simulink model "hexa_tilted_FxTESO_ANSFT"  (R2023a)
settings: Solver=ode4  StartTime=0.0  StopTime=72  FixedStep=0.01  RelTol=1e-3
model workspace (MAT data in the model file):
  hover_2m = [0  0  0  0  0  0; 0  0  0  0  0  0; 2  2  2  2  2  2; 0  0  0  0  0  0; 0  0  0  0  0  0; 0  0  0  0  0  0]
  square = [0  0  0  0  0  0; 0  0  0  0  0  0; 2.5  2.5  2.5  2.5  2.5  0; 0  0  0  0  0  0; 0  0  0  0  0  0; 0  0  0  0  0  0]
  tf = Simulink.Parameter
  tf.Value = 60
  tf.DataType = 'auto'
  tf.Complexity = 'real'
  tf.Dimensions = [1 1]
  tray0 = [0  0  0  0  0  0; 0  0  0  0  0  0; 0  5  5  5  5  0; 0  0  0  0  0  0; 0  0  0  0  0  0; 0  0  0  0  0  0]
  tray1 = [0  0  0  0  0  0; 0  0  0  0  0  0; 0  5  2.5  5  2.5  0; 0  0  0  0  0  0; 0  0  0  0  0  0; 0  0  0  0  0  0]
  tray2 = [0  2  2  -2  -2  0; 0  0  -2  -2  2  0; 0  5  2.5  5  2.5  0; 0  0  0  0  0  0; 0  0  0  0  0  0; 0  0  0  0  0  0]
  tray3 = [0  2  2  -2  -2  0; 0  0  -2  -2  2  0; 0  2.5  2.5  2.5  2.5  0; 0  0  0  0  0  0; 0  0  0  0  0  0; 0  0  0.785  0.785  0.785  0]
  tray4 = [0  2  2  -2  -2  0; 0  0  -2  -2  2  0; 0  5  2.5  5  2.5  0; 0  0.15  0.15  0.15  0.15  0; 0  0  0  0  0  0; 0  0  0.785  1.57  0.785  0]
  tray5 = [0  0  0  0  0  0; 0  0  0  0  0  0; 0  5  2.5  5  2.5  0; 0  0.15  0.15  0  0  0; 0  0  0.15  0.15  0  0; 0  0  0  0  0  0]
  tray_xyaw = [0  0  2  2  2  2; 0  0  0  0  0  0; 0  2.5  2.5  2.5  2.5  2.5; 0  0  0  0  0  0; 0  0  0  0  0  0; 1.57079632679  1.57079632679  1.57079632679  1.57079632679  1.57079632679  1.57079632679]
  tray_yaw = [0  0  0  0  0  0; 0  0  0  0  0  0; 0  2.5  5  2.5  0  2.5; 0  0  0  0  0  0; 0  0  0  0  0  0; 0  0  0.785  1.57  0.785  0]
undefined symbols (not defined in the file or in its folder): F, Light, MIL
libraries: dspsrcs4 x6, simulink x5, sharedtransform x2, robotcorelib x1, aerolibwind2 x1, SignalEditorBlockLib x1, uavutilslib x1
settings Model: Creator=adan  LastModifiedBy=adan
settings OptimizationCC: DefaultParameterBehavior=Inlined  EnhancedBackFolding=on  PassReuseOutputArgsAs=Individual arguments  ZeroExternalMemoryAtStartup=off  ZeroInternalMemoryAtStartup=off  OptimizeBlockOrder=speed  DifferentSizesBufferReuse=on  OptimizationCustomize=off  EfficientTunableParamExpr=on
settings DebuggingCC: ParameterTunabilityLossMsg=error
settings SFSimCC: MATLABDynamicMemAlloc=off
settings RTWCC: Description=Embedded Coder  SystemTargetFile=ert.tlc  TemplateMakefile=ert_default_tmf
settings CodeAppCC: ForceParamTrailComments=on  IgnoreCustomStorageClasses=off  OperatorAnnotations=on  SimulinkDataObjDesc=on  SFDataObjDesc=on  InsertBlockDesc=on
settings ERTTargetCC: TargetLangStandard=C99 (ISO)  GenerateSampleERTMain=on  InlinedParameterPlacement=NonHierarchical  ERTCustomFileTemplate=example_file_process.tlc

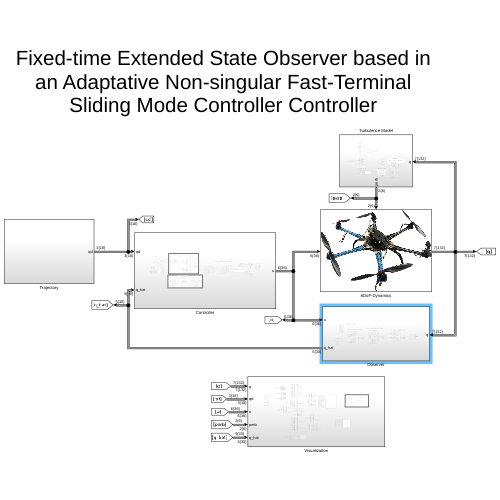
[thumbnail: Simulink's stored preview of the top-level diagram]
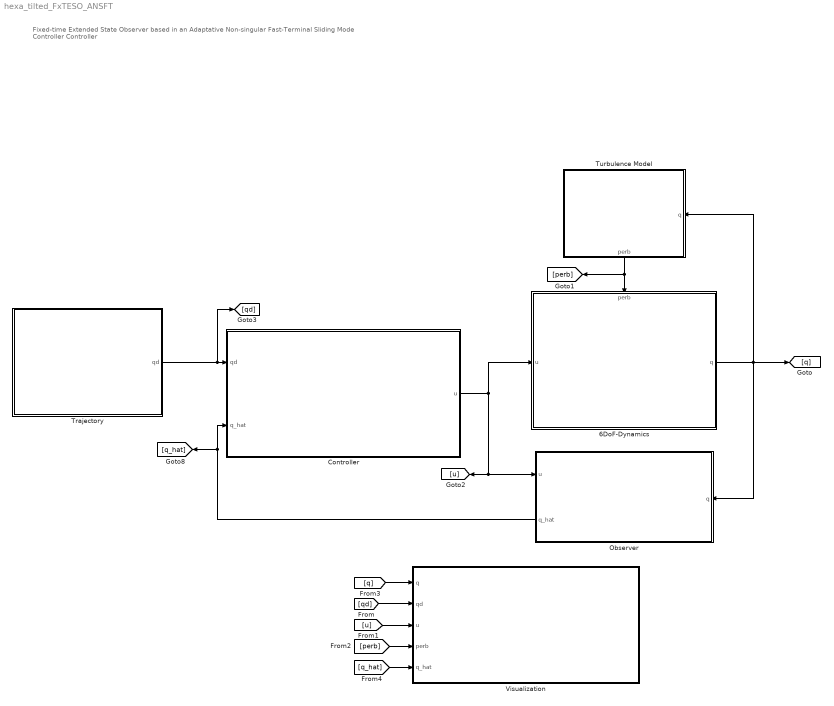
== system hexa_tilted_FxTESO_ANSFT ==
  note: Fixed-time Extended State Observer based in an Adaptative Non-singular Fast-Terminal Sliding Mode Controller Controller
  6DoF-Dynamics : Subsystem
      settings: PortSchema="{\"entries\":[{\"content\":{\"sides\":[{\"content\":{\"connectorIds\":[\"In1\"]},\"type\":\"ConnectorPlacement.EquallySpacedRectSide\",\"uuid\":\"d79ec49c-5563-41e0-ac59-6e897bc19fda\"},{\"content\":{\"connectorIds\":[\"Out1\"],\"side\":\"RIGHT\"},\"type\":\"ConnectorPlacement.EquallySpacedRectSide\",\"uuid\":\"1255043e-c90e-4bae-9fb4-4fa06f36f53e\"},{\"content\":{\"connectorIds\":[\"In2\"],\"side\":\"TOP\"},\"type\":\"ConnectorPlacement.EquallySpacedRectSide\",\"uuid\":\"823ada36-3f22-4ee3-87a1-180276f622bc\"}]},\"type\":\"ConnectorPlacement.EquallySpacedConnector\",\"uuid\":\"7403b609-b333-4977-a854-ed7a71f74338\"}],\"packageUris\":[\"http://schema.mathworks.com/mf0/Connector/R2020b\"],\"version\":\"1.0\"}"
      mask Display: image('$imagefile'); % Use "Edit Image" on toolstrip to change.
  Controller : Subsystem
  Observer : Subsystem
      settings: PortSchema="{\"entries\":[{\"content\":{\"sides\":[{\"content\":{\"connectorIds\":[\"In1\",\"Out1\"]},\"type\":\"ConnectorPlacement.EquallySpacedRectSide\",\"uuid\":\"d79ec49c-5563-41e0-ac59-6e897bc19fda\"},{\"content\":{\"connectorIds\":[\"In2\"],\"side\":\"RIGHT\"},\"type\":\"ConnectorPlacement.EquallySpacedRectSide\",\"uuid\":\"1255043e-c90e-4bae-9fb4-4fa06f36f53e\"},{\"content\":{\"side\":\"TOP\"},\"type\":\"ConnectorPlacement.EquallySpacedRectSide\",\"uuid\":\"823ada36-3f22-4ee3-87a1-180276f622bc\"}]},\"type\":\"ConnectorPlacement.EquallySpacedConnector\",\"uuid\":\"7403b609-b333-4977-a854-ed7a71f74338\"}],\"packageUris\":[\"http://schema.mathworks.com/mf0/Connector/R2020b\"],\"version\":\"1.0\"}"
  Trajectory : Subsystem
  Turbulence Model : Subsystem
      settings: PortSchema="{\"entries\":[{\"content\":{\"sides\":[{\"content\":{},\"type\":\"ConnectorPlacement.EquallySpacedRectSide\",\"uuid\":\"1a11629b-61d3-4a8e-8df8-8509e014e579\"},{\"content\":{\"connectorIds\":[\"In1\"],\"side\":\"RIGHT\"},\"type\":\"ConnectorPlacement.EquallySpacedRectSide\",\"uuid\":\"4b15c564-9714-4da5-9436-a08c0d95800f\"},{\"content\":{\"side\":\"TOP\"},\"type\":\"ConnectorPlacement.EquallySpacedRectSide\",\"uuid\":\"dd21b825-2def-4360-b27b-b8c6f475bfab\"},{\"content\":{\"connectorIds\":[\"Out1\"],\"side\":\"BOTTOM\"},\"type\":\"ConnectorPlacement.EquallySpacedRectSide\",\"uuid\":\"280c85e9-e29e-4357-9b86-73bf90833918\"}]},\"type\":\"ConnectorPlacement.EquallySpacedConnector\",\"uuid\":\"4c6e67eb-825c-4dd0-a48b-2afa68ae74f5\"}],\"packageUris\":[\"http://schema.mathworks.com/mf0/Connector/R2020b\"],\"version\":\"1.0\"}"
  Visualization : Subsystem
  wires:
  Trajectory/1(qd) -> [qd], Controller/1(qd)
  Controller/1(u) -> 6DoF-Dynamics/1(u), [u], Observer/1(u)
  6DoF-Dynamics/1(q) -> Turbulence Model/1(q), [q], Observer/2(q)
  Turbulence Model/1(perb) -> 6DoF-Dynamics/2(perb), [perb]
  Observer/1(q_hat) -> [q_hat], Controller/2(q_hat)
  [qd] -> Visualization/2(qd)
  [u] -> Visualization/3(u)
  [perb] -> Visualization/4(perb)
  [q_hat] -> Visualization/5(q_hat)
  [q] -> Visualization/1(q)

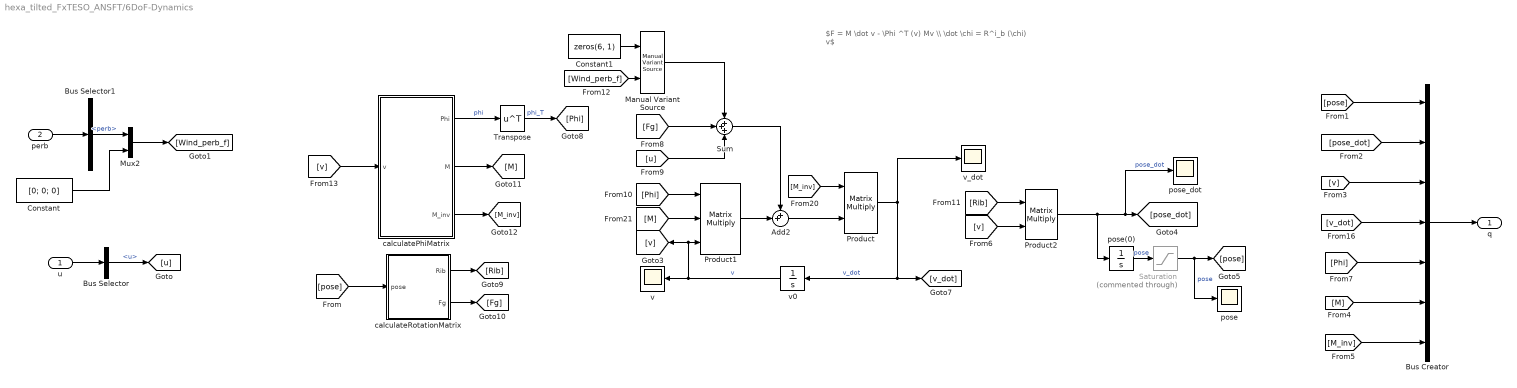
== system hexa_tilted_FxTESO_ANSFT/6DoF-Dynamics ==
  note: $F = M \dot v - \Phi ^T (v) Mv \\ \dot \chi = R^i_b (\chi) v$
  u : Inport
  perb : Inport  Port=2
  Add2 : Sum  Inputs=++|
  Bus Creator : BusCreator  Inputs=7
  Bus Selector : BusSelector  OutputSignals=u
  Bus Selector1 : BusSelector  OutputSignals=perb
  Constant : Constant  Value=[0; 0; 0]
  Constant1 : Constant  Value=zeros(6, 1)
  Manual Variant Source : simulink/Signal Routing/Manual Variant Source  NumChoices=2  LabelModeActiveChoice=V_2
  Mux2 : Mux  Inputs=2
  Product : Product  Multiplication=Matrix(*)
  Product1 : Product  Inputs=3  Multiplication=Matrix(*)
  Product2 : Product  Multiplication=Matrix(*)
  Saturation : Saturate  Commented=through  UpperLimit=[10, 10, 10, 10, 10, 10]'  LowerLimit=[-10, -10, 0, -10, -10, -10]'
  Sum : Sum  Inputs=+++
  Transpose : Math  Operator=transpose
  calculatePhiMatrix : MATLAB Function  TreatAsAtomicUnit=on
  calculateRotationMatrix : MATLAB Function  TreatAsAtomicUnit=on
  pose : Scope
  pose(0) : Integrator  InitialCondition=[0; 0; 0; 0; 0; 0]
  pose_dot : Scope
  v : Scope
  v0 : Integrator  InitialCondition=[0; 0; 0; 0; 0; 0]
  v_dot : Scope
  q : Outport
  wires:
  [M_inv] -> Product/1
  Product1/1 -> Add2/2
  [v] -> Product2/2
  Add2/1 -> Product/2
  Product/1 -> v_dot/1, [v_dot], v0/1  "v_dot"
  Product2/1 -> pose(0)/1, pose_dot/1, [pose_dot]  "pose_dot"
  [M] -> Product1/2
  [Rib] -> Product2/1
  [Phi] -> Product1/1
  [v] -> calculatePhiMatrix/1(v)
  calculatePhiMatrix/2(M) -> [M]
  calculatePhiMatrix/1(Phi) -> Transpose/1  "phi"
  calculatePhiMatrix/3(M_inv) -> [M_inv]
  Transpose/1 -> [Phi]  "phi_T"
  calculateRotationMatrix/1(Rib) -> [Rib]
  calculateRotationMatrix/2(Fg) -> [Fg]
  [pose] -> calculateRotationMatrix/1(pose)
  u/1 -> Bus Selector/1
  [pose] -> Bus Creator/1
  [pose_dot] -> Bus Creator/2
  [v] -> Bus Creator/3
  Bus Creator/1 -> q/1
  [Phi] -> Bus Creator/5
  [M] -> Bus Creator/6
  [M_inv] -> Bus Creator/7
  [Fg] -> Sum/2
  perb/1 -> Bus Selector1/1
  Bus Selector/1 -> [u]  "<u>"
  [u] -> Sum/3
  Bus Selector1/1 -> Mux2/1  "<perb>"
  Constant/1 -> Mux2/2
  Mux2/1 -> [Wind_perb_f]
  [Wind_perb_f] -> Manual Variant Source/2
  Sum/1 -> Add2/1
  v0/1 -> [v], Product1/3, v/1  "v"
  pose(0)/1 -> Saturation/1  "pose"
  [v_dot] -> Bus Creator/4
  Saturation/1 -> [pose], pose/1  "pose"
  Constant1/1 -> Manual Variant Source/1
  Manual Variant Source/1 -> Sum/1

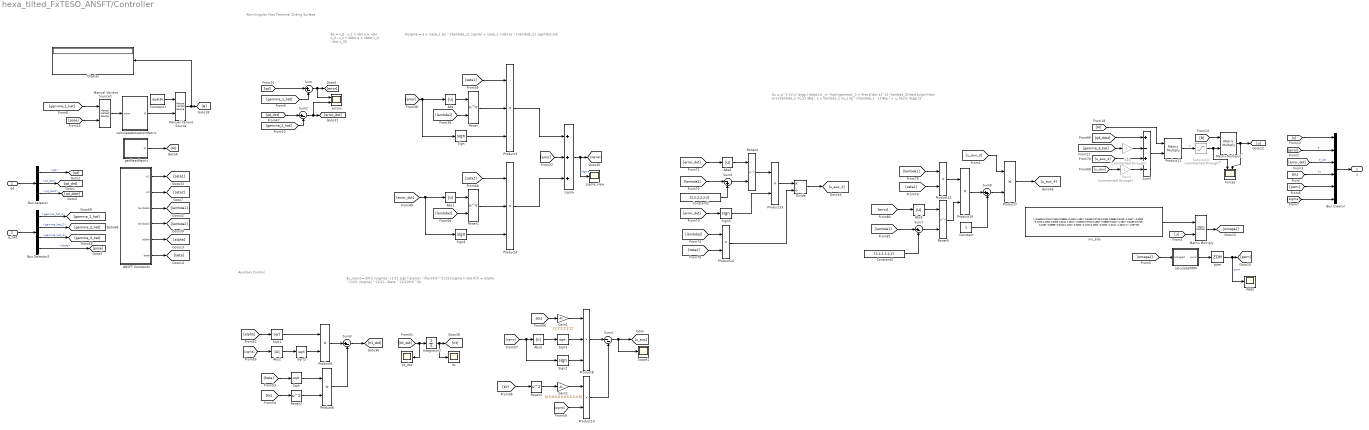
== system hexa_tilted_FxTESO_ANSFT/Controller ==
  note: $u = g^{-1}(x) \bigg [ \ddot{x}_d - \hat{\gamma}_3 + \frac{|\dot e|^{2- \lambda_2}\text{sign}(\dot e)}{\lambda_2 \xi_2} \Big ( 1 + \lambda_1 \xi_1 |e|^{\lambda_1 - 1}\Big ) + u_{aux} \bigg ]$
  note: Auxiliary Control
  note: Non-Singular Fast Terminal Sliding Surface
  note: $e = x_d - x_1 \\ \dot e = \dot x_d - x_2 \\ \ddot e = \ddot x_d - \dot x_2$
  note: $\sigma = e + \zeta_1 |e| ^{\lambda_1} sign(e) + \zeta_2 | \dot e| ^{\lambda_2} sign(\dot e)$
  note: $u_{aux}=-2K(t) |\sigma|^{1/2} sign (\sigma) - \frac{K(t)^2}{2}\sigma \\ \dot K(t) = \alpha ^{1/2} |\sigma| ^{1/2} - \beta ^{1/2}K(t)^2$
  qd : Inport
  q_hat : Inport  Port=2
  ANSFT Constants : MATLAB Function  TreatAsAtomicUnit=on
  Abs{,1..5} (6 alike) : Abs  SaturateOnIntegerOverflow=off
  Bus Creator : BusCreator  Inputs=6
  Bus Selector : BusSelector  OutputSignals=qd,qd_dot,qd_ddot
  Bus Selector2 : BusSelector  OutputSignals=gamma_hat_1,gamma_hat_2,gamma_hat_3,pose
  Constant : Constant
  Constant1 : Constant  Value=eye(6)
  Constant2 : Constant  Value=[2;2;2;2;2;2]
  Constant3 : Constant  Value=[1;1;1;1;1;1]
  Display : Display
  Divide : Product  Inputs=*/
  Forces : Scope  NumInputPorts=2
  Gain : Gain  Commented=through  Gain=-1
  Gain1 : Gain  Gain=[2;2;2;2;2;2]
  Gain2 : Gain  Gain=[0.5;0.5;0.5;0.5;0.5;0.5]
  Gain3 : Gain  Commented=through  Gain=-1
  Integrator2 : Integrator  InitialCondition=[0;0;0;0;0;0]
  Kt : Scope
  Kt_dot : Scope
  Manual Variant Source : simulink/Signal Routing/Manual Variant Source  NumChoices=2  LabelModeActiveChoice=V_2
  Manual Variant Source1 : simulink/Signal Routing/Manual Variant Source  NumChoices=2  LabelModeActiveChoice=V_2
  Matrix Multiply : Product  Multiplication=Matrix(*)
  Matrix Multiply1 : Product  Multiplication=Matrix(*)
  PWM : Scope
  Power{,1,4..5} (4 alike) : Math  Operator=pow
  Power2 : Math  Operator=square
  Power3 : Math  Operator=square
  Product{5..7,10,13..16} (8 alike) : Product
  Product11 : Product  Multiplication=Matrix(*)
  Product3 : Product  Inputs=3
  Product4 : Product  Inputs=3
  Product8 : Product  Inputs=3
  Saturation : Saturate  Commented=through  UpperLimit=[5, 5, 42, 0.5, 0.5, 0.5]'  LowerLimit=[-5, -5, 0, -0.5, -0.5, -0.5]'
  Scope1 : Scope
  Sign{,1..3} (4 alike) : Signum
  Sqrt{,1..3} (4 alike) : Sqrt
  Sum{,2..3,7} (4 alike) : Sum  Inputs=|+-
  Sum4 : Sum  Inputs=|--
  Sum5 : Sum  Inputs=+-+-
  Sum6 : Sum  Inputs=|-+
  Sum8 : Sum  Inputs=|++
  calculateActuationMatrix : MATLAB Function  TreatAsAtomicUnit=on
  calculatePWM : MATLAB Function  TreatAsAtomicUnit=on
  errors : Scope  NumInputPorts=2
  getMassMatrix : MATLAB Function  TreatAsAtomicUnit=on
  inv_allo : Constant  Value=|
      | [-0.6436    0.3716    0.1352    0.8869   -0.5120    1.1817;
      |             0.6436    0.3716    0.1352    0.8869    0.5120   -1.1817;
      |             -0.0000   -0.7431    0.1352    0.0000    1.0241    1.1817;
      |             -0.6436    0.3716    0.1352   -0.8869    0.5120   -1.1817;
      |             0.6436    0.3716    0.1352   -0.8869   -0.5120    1.1817;
      |             0.0000   -0.7431    0.1352   -0.0000   -1.0241   -1.1817;] * 1.0e+05;
  pwm : ZeroOrderHold  SampleTime=-1
  sigma : Sum  Inputs=+++
  sigma_view : Scope
  u : Outport
  wires:
  Product6/1 -> Sum3/2
  Sign1/1 -> Product4/3
  Sum8/1 -> Product7/2
  Product5/1 -> Sum3/1
  [error_dot] -> Abs4/1
  [u_aux_3] -> Product7/1
  Power5/1 -> Product16/2
  [zeta1] -> Product3/1
  Constant/1 -> Sum8/2
  Product16/1 -> Sum8/1
  Sqrt/1 -> Product6/1
  Product10/1 -> Sum4/2
  Sum6/1 -> Power4/2
  Product15/1 -> Product16/1
  [qd_ddot] -> Sum5/1
  [lambda2] -> Sum6/1
  Sum4/1 -> Scope1/1, [u_aux]
  [Kt] -> Power2/1
  Gain1/1 -> Product8/1
  Sum5/1 -> Product11/2
  Sqrt1/1 -> Product5/1
  Constant2/1 -> Sum6/2
  Sign3/1 -> Product13/2
  [lambda1] -> Sum7/1
  [gamma_2_hat] -> Sum2/2
  Power3/1 -> Gain2/1
  Product3/1 -> sigma/1
  [beta] -> Sqrt/1
  Abs4/1 -> Power4/1
  [Kt] -> Gain1/1
  [error_dot] -> Sign1/1, Abs1/1
  Divide/1 -> [u_aux_3]
  [sigma] -> Sign2/1, Abs3/1
  [zeta2] -> Product14/2
  Sum3/1 -> [Kt_dot]
  Product8/1 -> Sum4/1
  [sigma] -> Abs2/1
  Power/1 -> Product3/2
  Product4/1 -> sigma/3
  Constant3/1 -> Sum7/2
  [error] -> sigma/2
  Abs3/1 -> Sqrt3/1
  [alpha] -> Sqrt1/1
  Sum7/1 -> Power5/2
  Sqrt2/1 -> Product5/2
  Power4/1 -> Product13/1
  [M] -> Product11/1
  sigma/1 -> sigma_view/1, [sigma]  "sigma"
  Sign/1 -> Product3/3
  Abs2/1 -> Sqrt2/1
  [Kt_dot] -> Kt_dot/1, Integrator2/1
  Power1/1 -> Product4/2
  [lambda2] -> Product14/1
  Power2/1 -> Product6/2
  [zeta1] -> Product15/2
  [Kt] -> Power3/1
  [lambda1] -> Product15/1
  [error_dot] -> Sign3/1
  Sqrt3/1 -> Product8/2
  Product13/1 -> Divide/1
  [zeta2] -> Product4/1
  Integrator2/1 -> Kt/1, [Kt]
  [gamma_1_hat] -> Sum/2
  Abs/1 -> Power/1
  [qd] -> Sum/1
  Abs1/1 -> Power1/1
  Sum2/1 -> errors/2, [error_dot]
  Sum/1 -> errors/1, [error]
  Gain2/1 -> Product10/1
  Product14/1 -> Divide/2
  [lambda2] -> Power1/2
  [error] -> Abs5/1
  Abs5/1 -> Power5/1
  Product7/1 -> [u_aux_4]
  [sigma] -> Product10/2
  [lambda1] -> Power/2
  Sign2/1 -> Product8/3
  [error] -> Sign/1, Abs/1
  [qd_dot] -> Sum2/1
  Bus Creator/1 -> u/1
  ANSFT Constants/3(lambda1) -> [lambda1]
  ANSFT Constants/1(xi1) -> [zeta1]
  ANSFT Constants/2(xi2) -> [zeta2]
  ANSFT Constants/5(alpha) -> [alpha]
  ANSFT Constants/6(beta) -> [beta]
  ANSFT Constants/4(lambda2) -> [lambda2]
  qd/1 -> Bus Selector/1
  Bus Selector/2 -> [qd_dot]  "<qd_dot>"
  Bus Selector/1 -> [qd]  "<qd>"
  Bus Selector/3 -> [qd_ddot]  "<qd_ddot>"
  Product11/1 -> Saturation/1  "u"
  [error] -> Bus Creator/2  "e"
  [error_dot] -> Bus Creator/3  "e_dot"
  [Kt] -> Bus Creator/4  "kt"
  inv_allo/1 -> Matrix Multiply/1
  [u] -> Matrix Multiply/2
  Matrix Multiply/1 -> [omega2]
  [omega2] -> calculatePWM/1(omega2)
  calculatePWM/1(pwm) -> pwm/1
  pwm/1 -> PWM/1, [pwm]  "pwm"
  [pwm] -> Bus Creator/5
  [sigma] -> Bus Creator/6
  q_hat/1 -> Bus Selector2/1
  Bus Selector2/2 -> [gamma_2_hat]  "<gamma_hat_2>"
  Bus Selector2/3 -> [gamma_3_hat]  "<gamma_hat_3>"
  Bus Selector2/1 -> [gamma_1_hat]  "<gamma_hat_1>"
  [gamma_3_hat] -> Gain/1
  [u] -> Bus Creator/1
  Saturation/1 -> Matrix Multiply1/2, Forces/1  "u"
  getMassMatrix/1(M) -> [M]
  [u_aux_4] -> Sum5/3
  [u_aux] -> Gain3/1
  Gain/1 -> Sum5/2
  Gain3/1 -> Sum5/4
  calculateActuationMatrix/1(B) -> Manual Variant Source/2
  [gamma_1_hat] -> Manual Variant Source1/1
  Matrix Multiply1/1 -> Forces/2, [u]  "u"
  [B] -> Matrix Multiply1/1
  Manual Variant Source/1 -> Display/1, [B]
  Constant1/1 -> Manual Variant Source/1
  Bus Selector2/4 -> [pose]  "<pose>"
  Manual Variant Source1/1 -> calculateActuationMatrix/1(pose)
  [pose] -> Manual Variant Source1/2

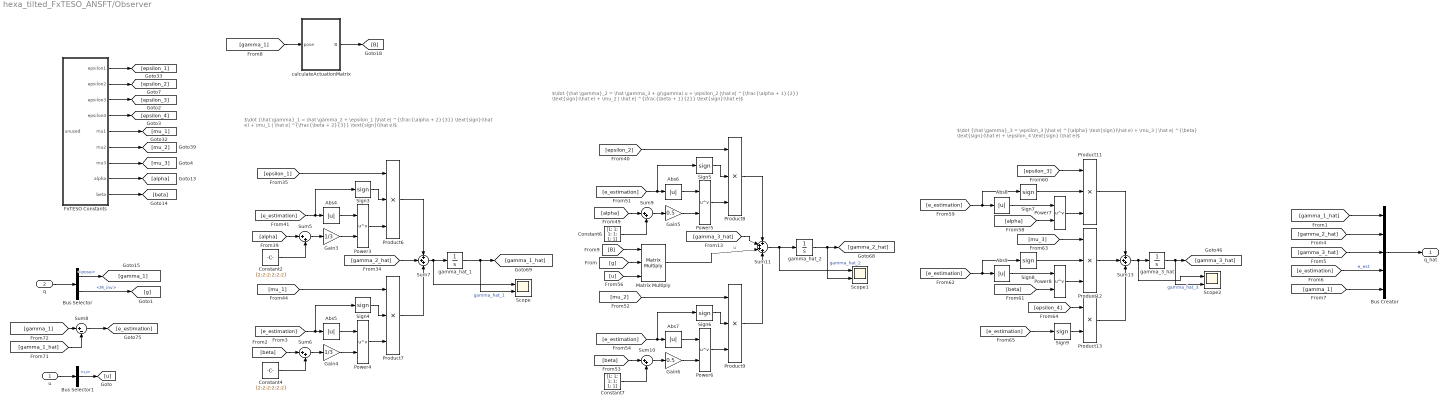
== system hexa_tilted_FxTESO_ANSFT/Observer ==
  note: $\dot {\hat \gamma}_3 = \epsilon_3 |\hat e| ^{\alpha} \text{sign}(\hat e) + \mu_3 | \hat e| ^{\beta} \text{sign}(\hat e) + \epsilon_4 \text{sign} (\hat e)$
  note: $\dot {\hat \gamma}_1 = \hat \gamma_2 + \epsilon_1 |\hat e| ^{\frac{\alpha + 2}{3}} \text{sign}(\hat e) + \mu_1 | \hat e| ^{\frac{\beta + 2}{3}} \text{sign}(\hat e)$
  note: $\dot {\hat \gamma}_2 = \hat \gamma_3 + g(\gamma) u + \epsilon_2 |\hat e| ^{\frac{\alpha + 1}{2}} \text{sign}(\hat e) + \mu_2 | \hat e| ^{\frac{\beta + 1}{2}} \text{sign}(\hat e)$
  u : Inport
  q : Inport  Port=2
  Abs{4..9} (6 alike) : Abs  SaturateOnIntegerOverflow=off
  Bus Creator : BusCreator  Inputs=5
  Bus Selector : BusSelector  OutputSignals=pose,M_inv
  Bus Selector1 : BusSelector  OutputSignals=u
  Constant2 : Constant  Value=[2;2;2;2;2;2]
  Constant4 : Constant  Value=[2;2;2;2;2;2]
  Constant6 : Constant  Value=[1; 1; 1; 1; 1; 1]
  Constant7 : Constant  Value=[1; 1; 1; 1; 1; 1]
  FxTESO Constants : MATLAB Function  TreatAsAtomicUnit=on
  Gain3 : Gain  Gain=1/3
  Gain4 : Gain  Gain=1/3
  Gain5 : Gain  Gain=0.5
  Gain6 : Gain  Gain=0.5
  Matrix Multiply : Product  Inputs=3  Multiplication=Matrix(*)
  Power{3..8} (6 alike) : Math  Operator=pow
  Product{6..9,11..12} (6 alike) : Product  Inputs=3
  Product13 : Product
  Scope : Scope  NumInputPorts=2
  Scope1 : Scope  NumInputPorts=2
  Scope2 : Scope  NumInputPorts=2
  Sign{3..9} (7 alike) : Signum
  Sum{5..6,9..10} (4 alike) : Sum  Inputs=|++
  Sum11 : Sum  Inputs=++++
  Sum13 : Sum  Inputs=+++
  Sum7 : Sum  Inputs=+++
  Sum8 : Sum  Inputs=|+-
  calculateActuationMatrix : MATLAB Function  TreatAsAtomicUnit=on
  gamma_3_hat : Integrator  InitialCondition=[0; 0; -9.81; 0; 0; 0]
  gamma_hat_1 : Integrator  InitialCondition=[0; 0; 0; 0; 0; 0]
  gamma_hat_2 : Integrator  InitialCondition=zeros(6,1)
  q_hat : Outport
  wires:
  [gamma_1] -> Sum8/1
  Gain6/1 -> Power6/2
  [alpha] -> Power7/2
  [gamma_3_hat] -> Sum11/2
  Sign7/1 -> Product11/2
  Sum7/1 -> Scope/1, gamma_hat_1/1
  Abs7/1 -> Power6/1
  [gamma_1_hat] -> Sum8/2
  [alpha] -> Sum5/1
  Sum8/1 -> [e_estimation]
  Power4/1 -> Product7/3
  [epsilon_3] -> Product11/1
  Power3/1 -> Product6/3
  Constant2/1 -> Sum5/2
  Abs9/1 -> Power8/1
  Sign5/1 -> Product8/2
  [e_estimation] -> Abs9/1, Sign8/1
  Gain4/1 -> Power4/2
  [e_estimation] -> Sign5/1, Abs6/1
  [mu_3] -> Product12/1
  Power7/1 -> Product11/3
  [beta] -> Power8/2
  Sign8/1 -> Product12/2
  [epsilon_1] -> Product6/1
  Bus Selector/1 -> [gamma_1]  "<pose>"
  Product13/1 -> Sum13/3
  Sign9/1 -> Product13/2
  Sum11/1 -> Scope1/1, gamma_hat_2/1
  Sum5/1 -> Gain3/1
  Product7/1 -> Sum7/3
  [e_estimation] -> Sign6/1, Abs7/1
  Abs4/1 -> Power3/1
  Abs8/1 -> Power7/1
  [e_estimation] -> Sign4/1, Abs5/1
  Sum9/1 -> Gain5/1
  [e_estimation] -> Abs8/1, Sign7/1
  Sum13/1 -> Scope2/1, gamma_3_hat/1
  [e_estimation] -> Sign3/1, Abs4/1
  Sign6/1 -> Product9/2
  [beta] -> Sum10/1
  Power8/1 -> Product12/3
  Sign3/1 -> Product6/2
  [mu_1] -> Product7/1
  [mu_2] -> Product9/1
  [gamma_2_hat] -> Sum7/2
  [epsilon_4] -> Product13/1
  [beta] -> Sum6/1
  Sum10/1 -> Gain6/1
  Gain3/1 -> Power3/2
  Constant4/1 -> Sum6/2
  gamma_hat_1/1 -> Scope/2, [gamma_1_hat]  "gamma_hat_1"
  [epsilon_2] -> Product8/1
  Abs5/1 -> Power4/1
  Sign4/1 -> Product7/2
  Gain5/1 -> Power5/2
  Product12/1 -> Sum13/2
  gamma_hat_2/1 -> Scope1/2, [gamma_2_hat]  "gamma_hat_2"
  Product6/1 -> Sum7/1
  [e_estimation] -> Sign9/1
  Product8/1 -> Sum11/1
  Constant6/1 -> Sum9/2
  [alpha] -> Sum9/1
  Abs6/1 -> Power5/1
  Power6/1 -> Product9/3
  Product11/1 -> Sum13/1
  Constant7/1 -> Sum10/2
  gamma_3_hat/1 -> Scope2/2, [gamma_3_hat]  "gamma_hat_3"
  Sum6/1 -> Gain4/1
  Power5/1 -> Product8/3
  Matrix Multiply/1 -> Sum11/3  "u"
  Product9/1 -> Sum11/4
  FxTESO Constants/5(mu1) -> [mu_1]
  FxTESO Constants/1(epsilon1) -> [epsilon_1]
  FxTESO Constants/2(epsilon2) -> [epsilon_2]
  FxTESO Constants/8(alpha) -> [alpha]
  FxTESO Constants/9(beta) -> [beta]
  FxTESO Constants/6(mu2) -> [mu_2]
  q/1 -> Bus Selector/1
  Bus Selector/2 -> [g]  "<M_inv>"
  FxTESO Constants/4(epsilon4) -> [epsilon_4]
  FxTESO Constants/3(epsilon3) -> [epsilon_3]
  FxTESO Constants/7(mu3) -> [mu_3]
  u/1 -> Bus Selector1/1
  Bus Selector1/1 -> [u]  "<u>"
  [gamma_1_hat] -> Bus Creator/1
  [gamma_3_hat] -> Bus Creator/3
  [gamma_2_hat] -> Bus Creator/2
  Bus Creator/1 -> q_hat/1
  [e_estimation] -> Bus Creator/4  "e_est"
  [gamma_1] -> Bus Creator/5
  [gamma_1] -> calculateActuationMatrix/1(pose)
  calculateActuationMatrix/1(B) -> [B]
  [B] -> Matrix Multiply/1
  [g] -> Matrix Multiply/2
  [u] -> Matrix Multiply/3

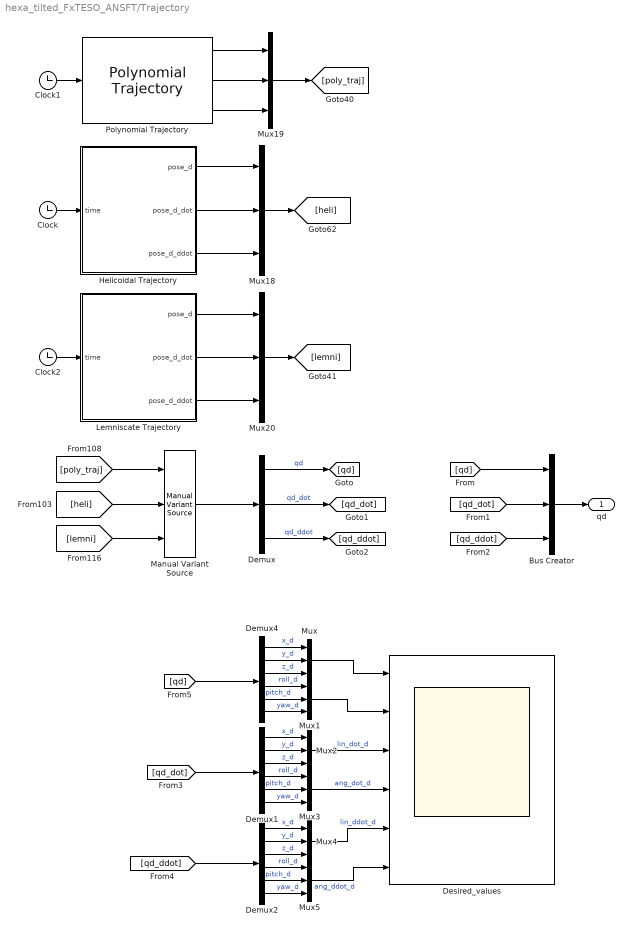
== system hexa_tilted_FxTESO_ANSFT/Trajectory ==
  Bus Creator : BusCreator  Inputs=3
  Clock : Clock
  Clock1 : Clock
  Clock2 : Clock
  Demux : Demux  Outputs=3
  Demux1 : Demux  Outputs=6
  Demux2 : Demux  Outputs=6
  Demux4 : Demux  Outputs=6
  Desired_values : Scope  NumInputPorts=6
  Helicoidal Trajectory : MATLAB Function  TreatAsAtomicUnit=on
  Lemniscate Trajectory : MATLAB Function  TreatAsAtomicUnit=on
  Manual Variant Source : simulink/Signal Routing/Manual Variant Source  NumChoices=3  LabelModeActiveChoice=V_2
  Mux{,1..5,18..20} (9 alike) : Mux  Inputs=3
  Polynomial Trajectory : robotcorelib/Polynomial Trajectory  WaypointSource=Internal  Waypoints=tray_xyaw  TimePoints=[ 0, 12, 24, 36, 48, tf ]  TimeInterval=[ 1, 4 ]  Method=Cubic Polynomial  ParameterSource=Internal  VelocityBoundaryCondition=zeros( 6, 6 )  AccelerationBoundaryCondition=zeros( 2, 5 )  SimulateUsing=Interpreted execution
  qd : Outport
  wires:
  Manual Variant Source/1 -> Demux/1
  Lemniscate Trajectory/2(pose_d_dot) -> Mux20/2
  [poly_traj] -> Manual Variant Source/1
  Polynomial Trajectory/3 -> Mux19/3
  Helicoidal Trajectory/1(pose_d) -> Mux18/1
  Clock1/1 -> Polynomial Trajectory/1
  Mux18/1 -> [heli]
  Lemniscate Trajectory/3(pose_d_ddot) -> Mux20/3
  Polynomial Trajectory/2 -> Mux19/2
  Demux/2 -> [qd_dot]  "qd_dot"
  Clock2/1 -> Lemniscate Trajectory/1(time)
  Helicoidal Trajectory/3(pose_d_ddot) -> Mux18/3
  Demux/1 -> [qd]  "qd"
  Mux19/1 -> [poly_traj]
  Mux20/1 -> [lemni]
  Lemniscate Trajectory/1(pose_d) -> Mux20/1
  Helicoidal Trajectory/2(pose_d_dot) -> Mux18/2
  Clock/1 -> Helicoidal Trajectory/1(time)
  Demux/3 -> [qd_ddot]  "qd_ddot"
  [heli] -> Manual Variant Source/2
  [lemni] -> Manual Variant Source/3
  Bus Creator/1 -> qd/1
  Polynomial Trajectory/1 -> Mux19/1
  Demux4/4 -> Mux1/1  "roll_d"
  Demux4/6 -> Mux1/3  "yaw_d"
  Demux4/3 -> Mux/3  "z_d"
  Demux4/2 -> Mux/2  "y_d"
  Demux4/1 -> Mux/1  "x_d"
  Demux4/5 -> Mux1/2  "pitch_d"
  [qd] -> Bus Creator/1
  [qd_dot] -> Bus Creator/2
  [qd_ddot] -> Bus Creator/3
  Demux1/6 -> Mux3/3  "yaw_d"
  Demux1/3 -> Mux2/3  "z_d"
  Demux1/5 -> Mux3/2  "pitch_d"
  [qd_dot] -> Demux1/1
  Demux1/1 -> Mux2/1  "x_d"
  Demux1/4 -> Mux3/1  "roll_d"
  Demux1/2 -> Mux2/2  "y_d"
  Demux2/6 -> Mux5/3  "yaw_d"
  Demux2/3 -> Mux4/3  "z_d"
  Demux2/5 -> Mux5/2  "pitch_d"
  [qd_ddot] -> Demux2/1
  Demux2/1 -> Mux4/1  "x_d"
  Demux2/4 -> Mux5/1  "roll_d"
  Demux2/2 -> Mux4/2  "y_d"
  Mux/1 -> Desired_values/1
  Mux1/1 -> Desired_values/2
  Mux2/1 -> Desired_values/3  "lin_dot_d"
  Mux3/1 -> Desired_values/4  "ang_dot_d"
  Mux4/1 -> Desired_values/5  "lin_ddot_d"
  Mux5/1 -> Desired_values/6  "ang_ddot_d"
  [qd] -> Demux4/1

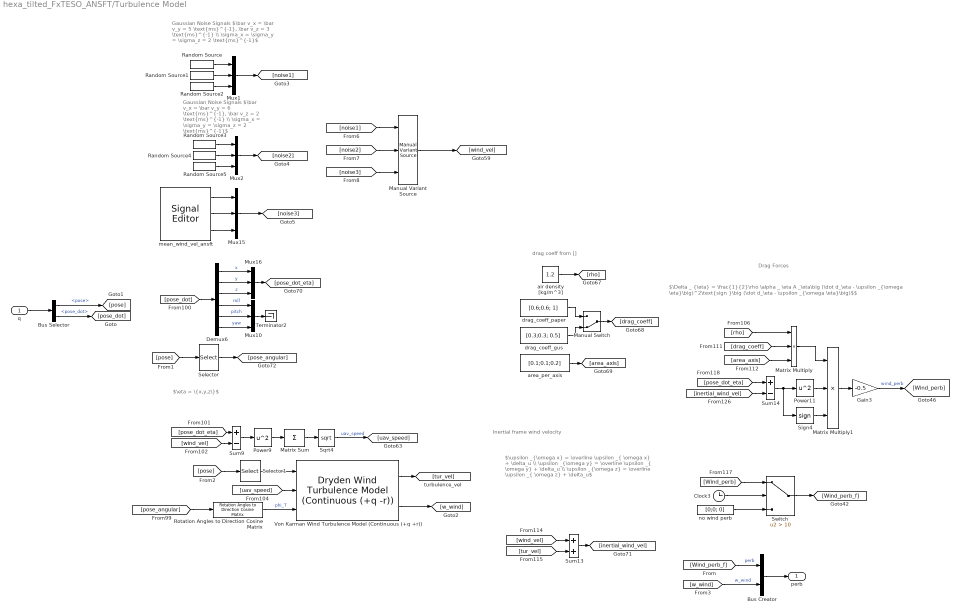
== system hexa_tilted_FxTESO_ANSFT/Turbulence Model ==
  note: $\Delta _ {\eta} = \frac{1}{2}\rho \alpha _ \eta A _\eta\big (\dot d_\eta - \upsilon _{\omega \eta}\big)^2\text{sign }\big (\dot d_\eta - \upsilon _{\omega \eta}\big)$$
  note: drag coeff from []
  note: $\upsilon _{\omega x} = \overline \upsilon _{ \omega x} + \delta_u \\ \upsilon _{\omega y} = \overline \upsilon _{ \omega y} + \delta_u \\ \upsilon _{\omega z} = \overline \upsilon _{ \omega z} + \delta_u$
  note: $\eta = \{x,y,z\}$
  note: Drag Forces
  note: Inertial frame wind velocity
  note: Gaussian Noise Signals
      | $\bar v_x = \bar v_y = 5 \text{ms}^{-1}, \bar v_z = 3 \text{ms}^{-1} \\ \sigma_x = \sigma_y = \sigma_z = 2 \text{ms}^{-1}$
  note: Gaussian Noise Signals
      | $\bar v_x = \bar v_y = 6 \text{ms}^{-1}, \bar v_z = 2 \text{ms}^{-1} \\ \sigma_x = \sigma_y = \sigma_z = 2 \text{ms}^{-1}$
  q : Inport
  Bus Creator : BusCreator  Inputs=2
  Bus Selector : BusSelector  OutputSignals=pose,pose_dot
  Clock3 : Clock
  Demux6 : Demux  Outputs=6
  Gain3 : Gain  Gain=-0.5
  Manual Variant Source : simulink/Signal Routing/Manual Variant Source  NumChoices=3  LabelModeActiveChoice=V_1
  Manual Switch : ManualSwitch  CurrentSetting=0
  Matrix Sum : Sum  Inputs=+
  Matrix Multiply : Product  Inputs=3
  Matrix Multiply1 : Product  Inputs=3
  Mux{1..2,10,15..16} (5 alike) : Mux  Inputs=3
  Power11 : Math  Operator=square
  Power9 : Math  Operator=square
  Random Source : dspsrcs4/Random Source  SrcType=Gaussian  NormMethod=Ziggurat  CltLength=12  MinVal=0  MaxVal=1  MeanVal=5  VarVal=2  RepMode=Not repeatable  rawSeed=1  IsInherit=off  SampMode=Discrete  SampTime=1  SampFrame=1  DataType=Double  OutComplex=Real  OutputFrames=off
  Random Source1 : dspsrcs4/Random Source  SrcType=Gaussian  NormMethod=Ziggurat  CltLength=12  MinVal=0  MaxVal=1  MeanVal=5  VarVal=2  RepMode=Not repeatable  rawSeed=1  IsInherit=off  SampMode=Discrete  SampTime=1  SampFrame=1  DataType=Double  OutComplex=Real  OutputFrames=off
  Random Source2 : dspsrcs4/Random Source  SrcType=Gaussian  NormMethod=Ziggurat  CltLength=12  MinVal=0  MaxVal=1  MeanVal=3  VarVal=2  RepMode=Not repeatable  rawSeed=1  IsInherit=off  SampMode=Discrete  SampTime=1  SampFrame=1  DataType=Double  OutComplex=Real  OutputFrames=off
  Random Source3 : dspsrcs4/Random Source  SrcType=Gaussian  NormMethod=Ziggurat  CltLength=12  MinVal=0  MaxVal=1  MeanVal=6  VarVal=2  RepMode=Not repeatable  rawSeed=1  IsInherit=off  SampMode=Discrete  SampTime=1  SampFrame=1  DataType=Double  OutComplex=Real  OutputFrames=off
  Random Source4 : dspsrcs4/Random Source  SrcType=Gaussian  NormMethod=Ziggurat  CltLength=12  MinVal=0  MaxVal=1  MeanVal=6  VarVal=2  RepMode=Not repeatable  rawSeed=1  IsInherit=off  SampMode=Discrete  SampTime=1  SampFrame=1  DataType=Double  OutComplex=Real  OutputFrames=off
  Random Source5 : dspsrcs4/Random Source  SrcType=Gaussian  NormMethod=Ziggurat  CltLength=12  MinVal=0  MaxVal=1  MeanVal=2  VarVal=2  RepMode=Not repeatable  rawSeed=1  IsInherit=off  SampMode=Discrete  SampTime=1  SampFrame=1  DataType=Double  OutComplex=Real  OutputFrames=off
  Rotation Angles to Direction Cosine Matrix : sharedtransform/Rotation Angles to Direction Cosine Matrix  rotationOrder=XYZ  aMode=aMode
  Selector : Selector  InputPortWidth=6  IndexOptions=Index vector (dialog)  Indices=[4:6]  OutputSizes=1
  Selector1 : Selector  InputPortWidth=6  IndexOptions=Index vector (dialog)  Indices=[3]  OutputSizes=1
  Sign4 : Signum
  Sqrt4 : Sqrt
  Sum13 : Sum
  Sum14 : Sum  Inputs=+-
  Sum9 : Sum  Inputs=+-
  Switch : Switch  Criteria=u2 > Threshold  Threshold=10  SaturateOnIntegerOverflow=off  InputSameDT=off
  Terminator2 : Terminator
  Von Karman Wind Turbulence Model (Continuous (+q +r)) : aerolibwind2/Dryden Wind Turbulence Model  (Continuous (+q -r))  units=Metric (MKS)  spec=MIL-F-8785C  model=Continuous Von Karman (+q -r)  W20=15  Wdeg=0  TurbProb=10^-2 - Light  L_high=762  Wingspan=10  ts=0.1  Seed=[23341 23342 23343 23344]  T_on=on
      settings: LibrarySourceBlock=|
      | aerolibwind2/Von Karman Wind Turbulence Model
      | (Continuous (+q +r))
  air density [kg/m^3] : Constant  Value=1.2
  area_per_axis : Constant  Value=[0.1;0.1;0.2]
  drag_coeff_gus : Constant  Value=[0.3;0.3; 0.5]
  drag_coeff_paper : Constant  Value=[0.6;0.6; 1]
  mean_wind_vel_ansft : SignalEditorBlockLib/Signal Editor  FileName=mean_wind_vel_ansft.mat  ActiveScenario=Velocidades_medias_del_viento  ActiveSignal=wean_wind_vel_x  IsBus=off  OutputBusObjectStr=Bus: BusObject  SampleTime=0  Interpolate=off  ZeroCross=off  OutputAfterFinalValue=Setting to zero  Unit=inherit  PreserveSignalName=on  ApplySigPropsToAllScenarios=on
  no wind perb : Constant  Value=[0;0; 0]
  perb : Outport
  wires:
  Demux6/1 -> Mux16/1  "x"
  [rho] -> Matrix Multiply/1
  Demux6/3 -> Mux16/3  "z"
  Manual Switch/1 -> [drag_coeff]
  Power11/1 -> Matrix Multiply1/2
  Von Karman Wind Turbulence Model (Continuous (+q +r))/1 -> [tur_vel]
  Rotation Angles to Direction Cosine Matrix/1 -> Von Karman Wind Turbulence Model (Continuous (+q +r))/3  "phi_T"
  drag_coeff_paper/1 -> Manual Switch/1
  Matrix Sum/1 -> Sqrt4/1
  Gain3/1 -> [Wind_perb]  "wind_perb"
  Matrix Multiply/1 -> Matrix Multiply1/1
  Selector/1 -> [pose_angular]
  Sum9/1 -> Power9/1
  no wind perb/1 -> Switch/3
  Mux16/1 -> [pose_dot_eta]
  Clock3/1 -> Switch/2
  Sum14/1 -> Sign4/1, Power11/1
  [area_axis] -> Matrix Multiply/3
  Von Karman Wind Turbulence Model (Continuous (+q +r))/2 -> [w_wind]
  [uav_speed] -> Von Karman Wind Turbulence Model (Continuous (+q +r))/2
  Demux6/4 -> Mux10/1  "roll"
  [drag_coeff] -> Matrix Multiply/2
  air density [kg/m^3]/1 -> [rho]
  Mux10/1 -> Terminator2/1
  area_per_axis/1 -> [area_axis]
  [pose_angular] -> Rotation Angles to Direction Cosine Matrix/1
  drag_coeff_gus/1 -> Manual Switch/2
  Sum13/1 -> [inertial_wind_vel]
  Switch/1 -> [Wind_perb_f]
  [pose_dot_eta] -> Sum9/1
  Demux6/5 -> Mux10/2  "pitch"
  [tur_vel] -> Sum13/2
  Selector1/1 -> Von Karman Wind Turbulence Model (Continuous (+q +r))/1
  [pose_dot_eta] -> Sum14/1
  [wind_vel] -> Sum9/2
  [Wind_perb] -> Switch/1
  [wind_vel] -> Sum13/1
  Sqrt4/1 -> [uav_speed]  "uav_speed"
  Demux6/6 -> Mux10/3  "yaw"
  Sign4/1 -> Matrix Multiply1/3
  Demux6/2 -> Mux16/2  "y"
  Power9/1 -> Matrix Sum/1
  Matrix Multiply1/1 -> Gain3/1
  [pose_dot] -> Demux6/1
  [inertial_wind_vel] -> Sum14/2
  Bus Creator/1 -> perb/1
  [Wind_perb_f] -> Bus Creator/1  "perb"
  q/1 -> Bus Selector/1
  Bus Selector/2 -> [pose_dot]  "<pose_dot>"
  Bus Selector/1 -> [pose]  "<pose>"
  [pose] -> Selector/1
  [pose] -> Selector1/1
  [w_wind] -> Bus Creator/2  "w_wind"
  mean_wind_vel_ansft/2 -> Mux15/2
  Mux2/1 -> [noise2]
  Manual Variant Source/1 -> [wind_vel]
  [noise2] -> Manual Variant Source/2
  Random Source4/1 -> Mux2/2
  mean_wind_vel_ansft/3 -> Mux15/3
  mean_wind_vel_ansft/1 -> Mux15/1
  Random Source/1 -> Mux1/1
  Mux1/1 -> [noise1]
  Random Source5/1 -> Mux2/3
  Random Source2/1 -> Mux1/3
  [noise3] -> Manual Variant Source/3
  Mux15/1 -> [noise3]
  Random Source3/1 -> Mux2/1
  Random Source1/1 -> Mux1/2
  [noise1] -> Manual Variant Source/1

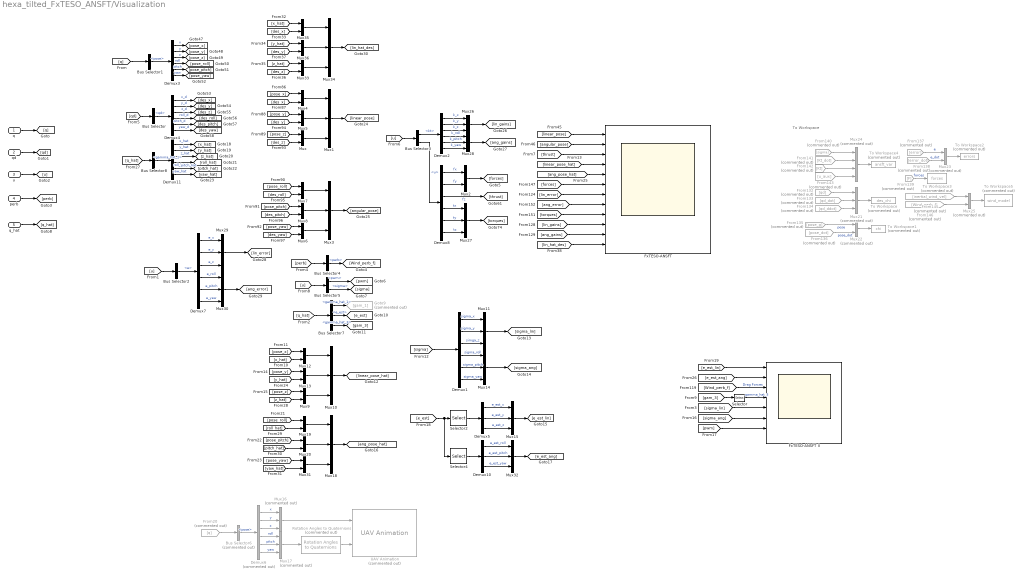
== system hexa_tilted_FxTESO_ANSFT/Visualization ==
  note: To Workspace
  q : Inport
  qd : Inport  Port=2
  u : Inport  Port=3
  perb : Inport  Port=4
  q_hat : Inport  Port=5
  Bus Selector : BusSelector  OutputSignals=qd
  Bus Selector1 : BusSelector  OutputSignals=pose
  Bus Selector2 : BusSelector  OutputSignals=e
  Bus Selector3 : BusSelector  OutputSignals=kt,u
  Bus Selector4 : BusSelector  OutputSignals=perb
  Bus Selector5 : BusSelector  OutputSignals=pwm,sigma
  Bus Selector6 : BusSelector  Commented=on  OutputSignals=pose
  Bus Selector7 : BusSelector  OutputSignals=gamma_hat_1,e_est,gamma_hat_3
  Bus Selector8 : BusSelector  OutputSignals=gamma_hat_1
  Demux{1..4,7..8,11} (7 alike) : Demux  Outputs=6
  Demux10 : Demux  Outputs=3
  Demux5 : Demux  Outputs=3
  Demux6 : Demux  Commented=on  Outputs=6
  From132 : From  Commented=on  GotoTag=qd
  From133 : From  Commented=on  GotoTag=qd_dot
  From134 : From  Commented=on  GotoTag=qd_ddot
  From135 : From  Commented=on  GotoTag=pose_g
  From136 : From  Commented=on  GotoTag=pose_dot
  From137 : From  Commented=on  GotoTag=error
  From138 : From  Commented=on  GotoTag=error_dot
  From139 : From  Commented=on  GotoTag=F
  From140 : From  Commented=on  GotoTag=sigma
  From141 : From  Commented=on  GotoTag=Kt_dot
  From142 : From  Commented=on  GotoTag=Kt
  From143 : From  Commented=on  GotoTag=u_aux
  From145 : From  Commented=on  GotoTag=inertial_wind_vel
  From146 : From  Commented=on  GotoTag=Wind_perb_f
  From20 : From  Commented=on  GotoTag=q
  FxTESO-ANSFT : Scope  NumInputPorts=12
  FxTESO-ANSFT II : Scope  NumInputPorts=8
  Goto9 : Goto  Commented=on  GotoTag=gam_1
  Mux{,2,4..9,12..13,19..20,31,33,35..36} (16 alike) : Mux  Inputs=2
  Mux{1,3,10..11,14..15,18,26..30,32,34} (14 alike) : Mux  Inputs=3
  Mux16 : Mux  Commented=on  Inputs=3
  Mux17 : Mux  Commented=on  Inputs=3
  Mux21 : Mux  Commented=on  Inputs=3
  Mux22 : Mux  Commented=on  Inputs=2
  Mux23 : Mux  Commented=on  Inputs=2
  Mux24 : Mux  Commented=on
  Mux25 : Mux  Commented=on  Inputs=2
  Rotation Angles to Quaternions : sharedtransform/Rotation Angles to Quaternions  Commented=on  rotationOrder=XYZ  aMode=aMode
  Selector : Selector  InputPortWidth=6  IndexOptions=Index vector (dialog)  Indices=[1:3]  OutputSizes=1
  Selector2 : Selector  InputPortWidth=6  IndexOptions=Index vector (dialog)  Indices=[1:3]  OutputSizes=1
  Selector4 : Selector  InputPortWidth=6  IndexOptions=Index vector (dialog)  Indices=[4:6]  OutputSizes=1
  To Workspace : ToWorkspace  Commented=on  VariableName=des_chi  SaveFormat=Structure With Time  SampleTime=-1
  To Workspace1 : ToWorkspace  Commented=on  VariableName=chi  SaveFormat=Structure With Time  SampleTime=-1
  To Workspace2 : ToWorkspace  Commented=on  VariableName=errors  SaveFormat=Structure With Time  SampleTime=-1
  To Workspace3 : ToWorkspace  Commented=on  VariableName=forces  SaveFormat=Structure With Time  SampleTime=-1
  To Workspace4 : ToWorkspace  Commented=on  VariableName=ansft_var  SaveFormat=Structure With Time  SampleTime=-1
  To Workspace5 : ToWorkspace  Commented=on  VariableName=wind_model  SaveFormat=Structure With Time  SampleTime=-1
  UAV Animation : uavutilslib/UAV Animation  Commented=on  UAVType=Multirotor  UAVSize=1  InertialZDirection=Up  SampleTime=-1
  wires:
  Demux2/2 -> Mux26/2  "k_y"
  From137/1 -> Mux23/1  "e"
  Mux6/1 -> Mux3/3
  Mux25/1 -> To Workspace5/1
  Mux26/1 -> [lin_gains]
  Demux3/4 -> [pose_roll]  "roll"
  From145/1 -> Mux25/1
  Demux8/3 -> [thrust]  "fz"
  Mux2/1 -> [forces]
  From143/1 -> Mux24/4
  From132/1 -> Mux21/1
  Demux7/5 -> Mux30/2  "e_pitch"
  From142/1 -> Mux24/3
  From140/1 -> Mux24/1
  From135/1 -> Mux22/1  "pose"
  Demux7/6 -> Mux30/3  "e_yaw"
  From136/1 -> Mux22/2  "pose_dot"
  Mux3/1 -> [angular_pose]
  Mux5/1 -> Mux1/2
  [pose_x] -> Mux4/1
  [pose_z] -> Mux/1
  Mux21/1 -> To Workspace/1
  Bus Selector7/2 -> [e_est]  "<e_est>"
  [Wind_perb_f] -> FxTESO-ANSFT II/3  "Drag Forces"
  Demux8/4 -> Mux27/1  "tx"
  Mux/1 -> Mux1/3
  Bus Selector1/1 -> Demux3/1  "<pose>"
  [q_hat] -> Bus Selector7/1
  Demux3/1 -> [pose_x]  "x"
  Bus Selector4/1 -> [Wind_perb_f]  "<perb>"
  Mux4/1 -> Mux1/1
  Demux7/3 -> Mux29/3  "e_z"
  From141/1 -> Mux24/2
  [des_pitch] -> Mux8/2
  [perb] -> Bus Selector4/1
  Demux4/5 -> [des_pitch]  "pitch_d"
  [gam_3] -> Selector/1
  Mux7/1 -> Mux3/1
  Demux4/2 -> [des_y]  "y_d"
  Demux8/2 -> Mux2/2  "fy"
  Demux2/3 -> Mux26/3  "k_z"
  [qd] -> Bus Selector/1
  Mux28/1 -> [ang_gains]
  [u] -> Bus Selector2/1
  [u] -> Bus Selector3/1
  Mux1/1 -> [linear_pose]
  Mux24/1 -> To Workspace4/1
  Demux3/3 -> [pose_z]  "z"
  Mux8/1 -> Mux3/2
  From133/1 -> Mux21/2
  Selector/1 -> FxTESO-ANSFT II/4  "gamma_hat_3"
  [u] -> Bus Selector5/1
  Mux22/1 -> To Workspace1/1
  Bus Selector3/2 -> Demux8/1  "<u>"
  Demux2/1 -> Mux26/1  "k_x"
  Mux30/1 -> [ang_error]
  [des_y] -> Mux5/2
  Demux2/4 -> Mux28/1  "k_roll"
  From139/1 -> To Workspace3/1  "forces"
  Bus Selector7/1 -> Goto9/1  "<gamma_hat_1>"
  [des_yaw] -> Mux6/2
  Mux27/1 -> [torques]
  Demux8/5 -> Mux27/2  "ty"
  From146/1 -> Mux25/2
  Bus Selector5/2 -> [sigma]  "<sigma>"
  Demux4/3 -> [des_z]  "z_d"
  Demux2/6 -> Mux28/3  "k_yaw"
  From138/1 -> Mux23/2  "e_dot"
  Demux3/6 -> [pose_yaw]  "yaw"
  Demux8/6 -> Mux27/3  "tz"
  Demux3/5 -> [pose_pitch]  "pitch"
  Demux4/1 -> [des_x]  "x_d"
  [pose_y] -> Mux5/1
  [des_x] -> Mux4/2
  Demux7/1 -> Mux29/1  "e_x"
  [linear_pose] -> FxTESO-ANSFT/1
  Demux8/1 -> Mux2/1  "fx"
  [pose_pitch] -> Mux8/1
  Mux29/1 -> [lin_error]
  [pose_yaw] -> Mux6/1
  [q] -> Bus Selector1/1
  [des_roll] -> Mux7/2
  Demux2/5 -> Mux28/2  "k_pitch"
  [pose_roll] -> Mux7/1
  Mux23/1 -> To Workspace2/1
  Demux4/4 -> [des_roll]  "roll_d"
  Demux3/2 -> [pose_y]  "y"
  Demux4/6 -> [des_yaw]  "yaw_d"
  Bus Selector3/1 -> Demux2/1  "<kt>"
  Bus Selector2/1 -> Demux7/1  "<e>"
  Demux7/2 -> Mux29/2  "e_y"
  Demux7/4 -> Mux30/1  "e_roll"
  Bus Selector7/3 -> [gam_3]  "<gamma_hat_3>"
  [des_z] -> Mux/2
  Bus Selector/1 -> Demux4/1  "<qd>"
  [angular_pose] -> FxTESO-ANSFT/2
  Bus Selector5/1 -> [pwm]  "<pwm>"
  From134/1 -> Mux21/3
  q/1 -> [q]
  qd/1 -> [qd]
  u/1 -> [u]
  perb/1 -> [perb]
  q_hat/1 -> [q_hat]
  Mux9/1 -> Mux10/3
  [pose_z] -> Mux9/1
  Mux10/1 -> [linear_pose_hat]
  Mux12/1 -> Mux10/1
  [pose_y] -> Mux13/1
  Mux13/1 -> Mux10/2
  [pose_x] -> Mux12/1
  Demux1/3 -> Mux11/3  "simga_z"
  Demux1/4 -> Mux14/1  "sigma_roll"
  Demux1/6 -> Mux14/3  "sigma_yaw"
  Demux1/2 -> Mux11/2  "sigma_y"
  [sigma] -> Demux1/1
  Mux11/1 -> [sigma_lin]
  Demux1/1 -> Mux11/1  "sigma_x"
  Demux1/5 -> Mux14/2  "sigma_pitch"
  Mux14/1 -> [sigma_ang]
  [sigma_lin] -> FxTESO-ANSFT II/5
  [sigma_ang] -> FxTESO-ANSFT II/6
  [pwm] -> FxTESO-ANSFT II/7
  [e_est] -> Selector4/1, Selector2/1
  Selector2/1 -> Demux5/1
  Demux5/3 -> Mux15/3  "e_est_z"
  Demux5/2 -> Mux15/2  "e_est_y"
  Demux5/1 -> Mux15/1  "e_est_x"
  Mux15/1 -> [e_est_lin]
  Demux6/2 -> Mux16/2  "y"
  Demux6/6 -> Mux17/3  "yaw"
  Demux6/5 -> Mux17/2  "pitch"
  Bus Selector6/1 -> Demux6/1  "<pose>"
  Demux6/4 -> Mux17/1  "roll"
  From20/1 -> Bus Selector6/1
  Demux6/3 -> Mux16/3  "z"
  Demux6/1 -> Mux16/1  "x"
  Mux17/1 -> Rotation Angles to Quaternions/1
  Rotation Angles to Quaternions/1 -> UAV Animation/2
  Mux16/1 -> UAV Animation/1
  [pose_roll] -> Mux19/1
  Mux31/1 -> Mux18/3
  [pose_yaw] -> Mux31/1
  Mux18/1 -> [ang_pose_hat]
  Mux19/1 -> Mux18/1
  [pose_pitch] -> Mux20/1
  Mux20/1 -> Mux18/2
  [thrust] -> FxTESO-ANSFT/3
  [linear_pose_hat] -> FxTESO-ANSFT/4
  [ang_pose_hat] -> FxTESO-ANSFT/5
  [forces] -> FxTESO-ANSFT/6
  [lin_error] -> FxTESO-ANSFT/7
  [ang_error] -> FxTESO-ANSFT/8
  [torques] -> FxTESO-ANSFT/9
  [lin_gains] -> FxTESO-ANSFT/10
  [ang_gains] -> FxTESO-ANSFT/11
  [e_est_lin] -> FxTESO-ANSFT II/1
  Selector4/1 -> Demux10/1
  Demux10/3 -> Mux32/3  "e_est_yaw"
  Demux10/1 -> Mux32/1  "e_est_roll"
  Demux10/2 -> Mux32/2  "e_est_pitch"
  Mux32/1 -> [e_est_ang]
  [e_est_ang] -> FxTESO-ANSFT II/2
  Demux11/3 -> [z_hat]  "z_hat"
  Demux11/1 -> [x_hat]  "x_hat"
  Demux11/6 -> [yaw_hat]  "yaw_hat"
  Bus Selector8/1 -> Demux11/1  "<gamma_hat_1>"
  Demux11/4 -> [roll_hat]  "roll_hat"
  Demux11/5 -> [pitch_hat]  "pitch_hat"
  Demux11/2 -> [y_hat]  "y_hat"
  [q_hat] -> Bus Selector8/1
  [x_hat] -> Mux12/2
  [y_hat] -> Mux13/2
  [z_hat] -> Mux9/2
  [roll_hat] -> Mux19/2
  [pitch_hat] -> Mux20/2
  [yaw_hat] -> Mux31/2
  [y_hat] -> Mux36/1
  [des_y] -> Mux36/2
  Mux36/1 -> Mux34/2
  [z_hat] -> Mux33/1
  [x_hat] -> Mux35/1
  [des_x] -> Mux35/2
  [des_z] -> Mux33/2
  Mux35/1 -> Mux34/1
  Mux33/1 -> Mux34/3
  Mux34/1 -> [lin_hat_des]
  [lin_hat_des] -> FxTESO-ANSFT/12

== matlab function hexa_tilted_FxTESO_ANSFT/Controller/getMassMatrix ==
  data: M output
function M  = fcn

m = 2.0; 
Jxx =  24778420.82/(1000*1000000); % kg m²
Jyy = 42217933.96/(1000*1000000); % kg m²
Jzz = 23948304.24/(1000*1000000); % kg m²

M = [m, 0, 0, 0, 0, 0;
    0, m, 0, 0, 0, 0;
    0, 0, m, 0, 0, 0;
    0, 0, 0, Jxx, 0, 0;
    0, 0, 0, 0, Jyy, 0;
    0, 0, 0, 0, 0, Jzz];

% M_inv = inv(M);

== matlab function hexa_tilted_FxTESO_ANSFT/Trajectory/Helicoidal Trajectory ==
  data: time input; pose_d output; pose_d_dot output; pose_d_ddot output
function [pose_d, pose_d_dot, pose_d_ddot]= fcn(time)

% pos_z = time / 12;
f = 0.15;
arg = f * (time - 5);
r = 2;

% hover for 5 s | include inclination in roll
% 5 metros al menos

roll = 0;
% yaw = pi / 2;
% yaw = 0;

if (time < 5)
    pos_x = 0;
    pos_y = 0;
    % roll = 0;
    pos_z = 0.4 * time;
    yaw = 0;
else
    pos_x = -r + r * cos (arg);
    pos_y = r * sin (arg);
    pos_z = 2;
    % roll = 0.15;
    yaw = (time - 5) * 2 * pi / 180; 
end

pose_d = [pos_x;
          pos_y;
          pos_z;
          roll;
          0;
          yaw];

% pos_z_dot = 1 / 12;
% yaw_dot = 0;

% hover for 5 s
if (time < 5)
    pos_x_dot = 0;
    pos_y_dot = 0;
    pos_z_dot = 0.4;
    yaw_dot = 0;
else
    pos_x_dot = - f * r * sin(arg);
    pos_y_dot = f * r * cos(arg);
    pos_z_dot = 0;
    yaw_dot = 2 * pi / 180;
end

pose_d_dot = [pos_x_dot;
              pos_y_dot;
              pos_z_dot;
              0;
              0;
              yaw_dot];

pos_z_ddot = 0;
% hover for 5 s
if (time < 5)
    pos_x_ddot = 0;
    pos_y_ddot = 0;
else
    pos_x_ddot = - f * f * r * cos(arg);
    pos_y_ddot = - f * f * r * sin(arg);
end

pose_d_ddot = [pos_x_ddot;
               pos_y_ddot;
               pos_z_ddot;
               0;
               0;
               0];

== matlab function hexa_tilted_FxTESO_ANSFT/Controller/ANSFT Constants ==
  data: xi1 output; xi2 output; lambda1 output; lambda2 output; alpha output; beta output
function [xi1, xi2, lambda1, lambda2, alpha, beta] = fcn

%% Constantes de la Superficie deslizante
% valores de zeta1 y zeta2
% zeta1 parecido a una ganancia proporcional
xi1 = [1; 1; 0.1; 1; 1; 5];

%zeta2 parecido a una ganancia derivatida
xi2 = [1.25; 1.25; 2; 0.5; 0.5; 0.5];

% lambda 1 > lambda2
lambda1 = [1.5; 1.5; 2; 1.5; 1.5; 5];

% 1 < lambda2 < 2
lambda2 = [1.2; 1.2; 1.25; 1.3; 1.3; 1.3];

%% Constantes del control auxiliar

%minimize sigma
alpha = [0.01; 0.01; 5; 16; 16; 10];

%aumetnar control, aumentar energía del sistema
beta = [8; 8; 0.5; 9; 9; 1];

== matlab function hexa_tilted_FxTESO_ANSFT/6DoF-Dynamics/calculatePhiMatrix ==
  data: Phi output; M output; M_inv output; v input
function [Phi, M, M_inv] = fcn(v)

%% system constants
m = 2.0; %5 mass 2.2 kg

Jxx =  24778420.82/(1000*1000000); % kg m²
Jyy = 42217933.96/(1000*1000000); % kg m²
Jzz = 23948304.24/(1000*1000000); % kg m²
%% Phi matrix calculation
uu = v(1);
vv = v(2);
ww = v(3);
pp = v(4);
qq = v(5);
rr = v(6);


Phi = [0, -rr, qq, 0, -ww, vv;
        rr, 0, -pp , ww, 0, -uu;
        -qq, pp, 0,  -vv, uu, 0;
        0, 0, 0, 0, -rr, qq; 
        0, 0, 0, rr, 0, -pp;
        0, 0, 0, -qq, pp, 0];

M = [m, 0, 0, 0, 0, 0;
    0, m, 0, 0, 0, 0;
    0, 0, m, 0, 0, 0;
    0, 0, 0, Jxx, 0, 0;
    0, 0, 0, 0, Jyy, 0;
    0, 0, 0, 0, 0, Jzz];

M_inv = inv(M);

== matlab function hexa_tilted_FxTESO_ANSFT/Trajectory/Lemniscate Trajectory ==
  data: time input; pose_d output; pose_d_dot output; pose_d_ddot output
function [pose_d, pose_d_dot, pose_d_ddot]= fcn(time)

%% Positions

arg = time / 4;

pos_x = cos(arg) ./ (1 + sin(arg) .* sin(arg));
pos_y = cos(arg) .* sin(arg) ./ (1 + sin(arg) .* sin(arg));
pos_z = time / 12;

yaw = time * 0;

pose_d = [pos_x;
          pos_y;
          pos_z;
          0;
          0;
          yaw];

%% Velocities

pos_z_dot = 1 / 12;
pos_x_dot = 0;
pos_y_dot = 0;
yaw_dot = 0;

pose_d_dot = [pos_x_dot;
              pos_y_dot;
              pos_z_dot;
              0;
              0;
              yaw_dot];

%% Accelerations

pos_z_ddot = 0;
pos_x_ddot = 0;
pos_y_ddot = 0;
yaw_ddot = 0;

pose_d_ddot = [pos_x_ddot;
               pos_y_ddot;
               pos_z_ddot;
               0;
               0;
               yaw_ddot];

== matlab function hexa_tilted_FxTESO_ANSFT/6DoF-Dynamics/calculateRotationMatrix ==
  data: pose input; Rib output; Fg output
function [Rib, Fg] = fcn(pose)

roll = pose(4);
pitch = pose(5);
yaw = pose(6);

m = 2.0; %5 mass 2.2 kg
g = -9.81; % gravity m/s²

R1 = [cos(yaw)*cos(pitch), -cos(roll)*sin(yaw) + cos(yaw)*sin(roll)*sin(pitch), sin(roll)*sin(yaw) + cos(roll)*cos(yaw)*sin(pitch);
       cos(pitch)*sin(yaw), cos(roll)*cos(yaw) + sin(yaw)*sin(pitch)*sin(roll), -cos(yaw)*sin(roll) + sin(yaw)*sin(pitch)*cos(roll);
       -sin(pitch), cos(pitch)*sin(roll), cos(pitch)*cos(roll)];

R2 = [1, sin(roll)*tan(pitch), cos(roll)*tan(pitch);
      0, cos(roll), -sin(roll);
      0, sin(roll)/cos(pitch), cos(roll)/cos(pitch)];

Rzeros = zeros(3);

Rib = [R1, Rzeros;
       Rzeros, R2];

%% Fg matrix calculation

Fg = [-m*g*sin(pitch);
      m*g*cos(pitch)*sin(roll);
      m*g*cos(pitch)*cos(roll);
      0;
      0;
      0];

% Fg = -Fg;

== matlab function hexa_tilted_FxTESO_ANSFT/Controller/calculatePWM ==
  data: omega2 input; pwm output
function pwm = fcn(omega2)

pwm = -1.3121e-09 .* omega2 .* omega2 + 0.00208 .* omega2 + 1107.922;

== matlab function hexa_tilted_FxTESO_ANSFT/Observer/FxTESO Constants ==
  data: unused input; epsilon1 output; epsilon2 output; epsilon3 output; epsilon4 output; mu1 output; mu2 output; mu3 output; alpha output; beta output
function [epsilon1, epsilon2, epsilon3, epsilon4, mu1, mu2, mu3, alpha, beta] = fcn(~)

epsilon1 = [16; 16; 16; 16; 16; 16];
epsilon2 = [60; 60; 60; 150; 150; 150];
epsilon3 = [100; 100; 100; 450; 450; 450];

epsilon4 = [0.01, 0.01, 0.01, 0.01, 0.01, 0.01]';

mu1 = epsilon1;
mu2 = epsilon2;
mu3 = epsilon3;

alpha = [0.6; 0.6; 0.6; 0.6; 0.6; 0.6];

beta = [1.2; 1.2; 1.2; 1.2; 1.2; 1.2];

%% Second set of parameters
% from 

% epsilon1 = [16; 16; 16; 16; 16; 16];
% epsilon2 = [150; 150; 150; 150; 150; 150];
% epsilon3 = [450; 450; 450; 450; 450; 450];
% 
% epsilon4 = [0.1, 0.1, 0.1, 0.01, 0.01, 0.01]';
% 
% mu1 = epsilon1;
% mu2 = epsilon2;
% mu3 = epsilon3;
% 
% alpha = [0.6; 0.6; 0.6; 0.6; 0.6; 0.6];
% 
% beta = [1.2; 1.2; 1.2; 1.2; 1.2; 1.2];

== matlab function hexa_tilted_FxTESO_ANSFT/Controller/calculateActuationMatrix ==
  data: pose input; B output
function B  = fcn(pose)

roll = pose(4);
pitch = pose(5);
yaw = pose(6);

R1 = [cos(yaw)*cos(pitch), -cos(roll)*sin(yaw) + cos(yaw)*sin(roll)*sin(pitch), sin(roll)*sin(yaw) + cos(roll)*cos(yaw)*sin(pitch);
       cos(pitch)*sin(yaw), cos(roll)*cos(yaw) + sin(yaw)*sin(pitch)*sin(roll), -cos(yaw)*sin(roll) + sin(yaw)*sin(pitch)*cos(roll);
       -sin(pitch), cos(pitch)*sin(roll), cos(pitch)*cos(roll)];

R2 = [1, sin(roll)*tan(pitch), cos(roll)*tan(pitch);
      0, cos(roll), -sin(roll);
      0, sin(roll)/cos(pitch), cos(roll)/cos(pitch)];

Rzeros = zeros(3);

B = [transpose(R1), Rzeros;
     Rzeros, inv(R2)];

== matlab function hexa_tilted_FxTESO_ANSFT/Observer/calculateActuationMatrix ==
  data: pose input; B output
function B  = fcn(pose)

roll = pose(4);
pitch = pose(5);
yaw = pose(6);

R1 = [cos(yaw)*cos(pitch), -cos(roll)*sin(yaw) + cos(yaw)*sin(roll)*sin(pitch), sin(roll)*sin(yaw) + cos(roll)*cos(yaw)*sin(pitch);
       cos(pitch)*sin(yaw), cos(roll)*cos(yaw) + sin(yaw)*sin(pitch)*sin(roll), -cos(yaw)*sin(roll) + sin(yaw)*sin(pitch)*cos(roll);
       -sin(pitch), cos(pitch)*sin(roll), cos(pitch)*cos(roll)];

R2 = [1, sin(roll)*tan(pitch), cos(roll)*tan(pitch);
      0, cos(roll), -sin(roll);
      0, sin(roll)/cos(pitch), cos(roll)/cos(pitch)];

Rzeros = zeros(3);

% B = [transpose(R1), Rzeros;
%      Rzeros, inv(R2)];

B = [R1, Rzeros;
     Rzeros, R2];
